simulink model "mass_spring_damper"  (R2022a)
settings: Solver=ode4  StartTime=0.0  StopTime=100  FixedStep=0.001  RelTol=1e-3
values from neighbouring files (symbols this model uses):
  b = 10    [mass_spring_damper_params_setup.m]
  F = 10    [mass_spring_damper_params_setup.m]
  k = 40    [mass_spring_damper_params_setup.m]
  M = 100    [mass_spring_damper_params_setup.m]
settings Model: Creator=stakk  LastModifiedBy=stakk

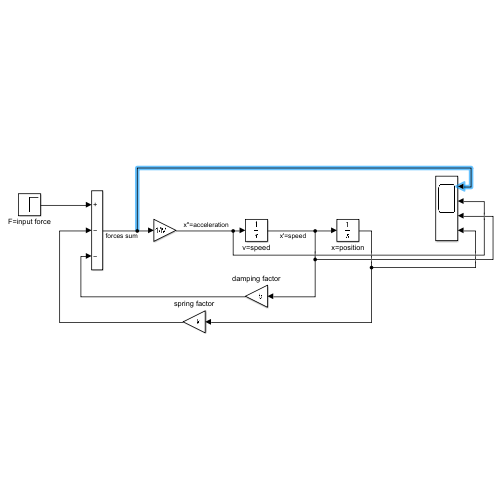
[thumbnail: Simulink's stored preview of the top-level diagram]
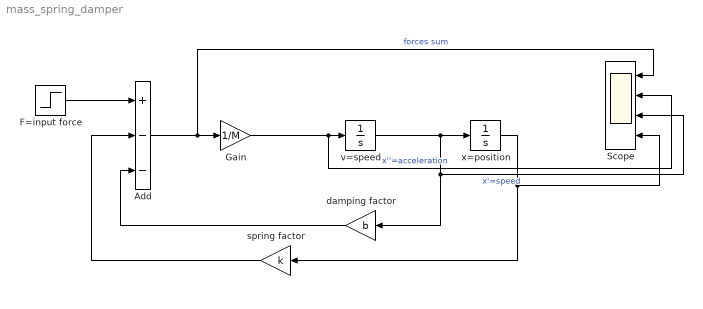
== system mass_spring_damper ==
  Add : Sum  Inputs=+--
  F=input force : Step  After=F  SampleTime=0
  Gain : Gain  Gain=1/M
  Scope : Scope  NumInputPorts=4
  damping factor : Gain  Gain=b
  spring factor : Gain  Gain=k
  v=speed : Integrator
  x=position : Integrator
  wires:
  Gain/1 -> Scope/2, v=speed/1  "x''=acceleration"
  v=speed/1 -> Scope/3, damping factor/1, x=position/1  "x'=speed"
  x=position/1 -> Scope/4, spring factor/1
  F=input force/1 -> Add/1
  damping factor/1 -> Add/3
  spring factor/1 -> Add/2
  Add/1 -> Scope/1, Gain/1  "forces sum"
